simulink model "milestoneone_mdl"  (R2024b)
settings: Solver=FixedStepAuto  StartTime=0.0  StopTime=10  FixedStep=1e-3  RelTol=1e-3  EnableMultiTasking=on
model workspace (MAT data in the model file):
  Var = 0
settings Model: ExtModeTrigDuration=5  Creator=alber  LastModifiedBy=alber
settings OptimizationCC: DefaultParameterBehavior=Inlined  EnhancedBackFolding=on  PassReuseOutputArgsAs=Individual arguments  ZeroExternalMemoryAtStartup=off  ZeroInternalMemoryAtStartup=off  MaxStackSize=64  OptimizeBlockOrder=speed  DifferentSizesBufferReuse=on  OptimizationCustomize=off  EfficientTunableParamExpr=on
settings DebuggingCC: ParameterTunabilityLossMsg=error
settings HardwareCC: ProdBitPerPointer=32  ProdBitPerSizeT=32  ProdBitPerPtrDiffT=32  ProdLargestAtomicInteger=Long  ProdLargestAtomicFloat=Double  ProdWordSize=32  ProdHWDeviceType=ARM Compatible->ARM Cortex
settings SFSimCC: MATLABDynamicMemAlloc=off
settings RTWCC: Description=Embedded Coder  SystemTargetFile=ert.tlc  HardwareBoard=NXP FRDM-K64F  TLCOptions="-aInlineSetEventsForThisBaseRateFcn=TLC_FALSE -aSuppressMultiTaskScheduler=TLC_FALSE  -aRateBasedStepFcn=0"  TemplateMakefile=ert_default_tmf  Toolchain=GNU Tools for ARM Embedded Processors
settings CodeAppCC: ForceParamTrailComments=on  IgnoreCustomStorageClasses=off  OperatorAnnotations=on  SimulinkDataObjDesc=on  SFDataObjDesc=on  InsertBlockDesc=on
settings ERTTargetCC: ExtModeTransport=4  ExtModeMexFile=sendToCommService
settings ConfigComp: CovBoundaryAbsTol=1.0e-5

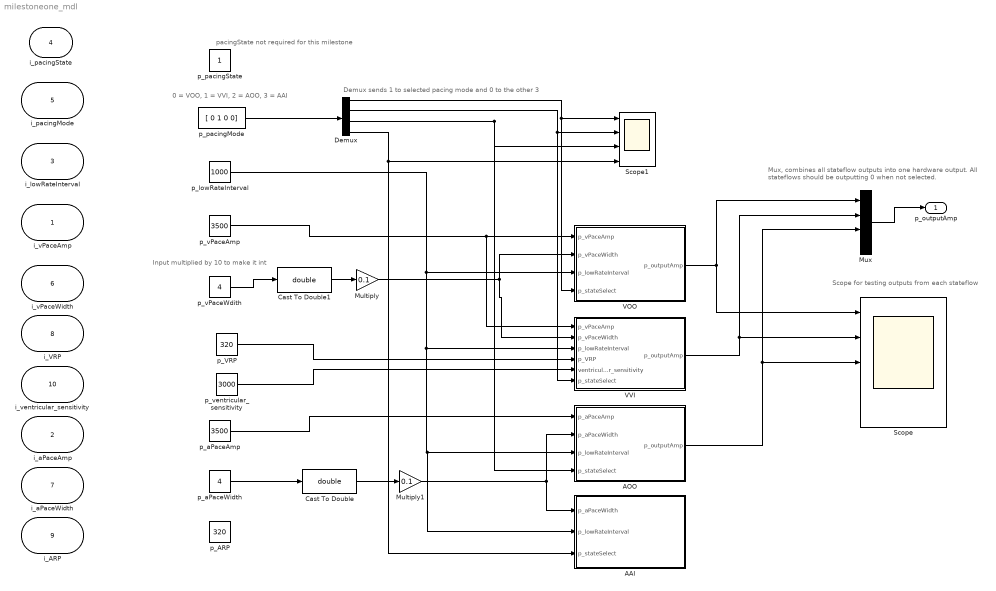
== system milestoneone_mdl ==
  note: pacingState not required for this milestone
  note: Demux sends 1 to selected pacing mode and 0 to the other 3
  note: Input multiplied by 10 to make it int
  note: 0 = VOO, 1 = VVI, 2 = AOO, 3 = AAI
  note: Scope for testing outputs from each stateflow
  note: Mux, combines all stateflow outputs into one hardware output.
      | All stateflows should be outputting 0 when not selected.
  i_vPaceAmp : Inport  OutMin=[500]  OutMax=[7000]  OutDataTypeStr=uint16  Unit=mV  PortDimensions=1
  i_aPaceAmp : Inport  Port=2  OutDataTypeStr=uint16  Unit=mV  PortDimensions=1
  i_lowRateInterval : Inport  Port=3  OutMin=[343]  OutMax=[2000]  OutDataTypeStr=uint16  Unit=Msec  PortDimensions=1
  i_pacingState : Inport  Port=4
  i_pacingMode : Inport  Port=5  OutDataTypeStr=uint8  PortDimensions=1
  i_vPaceWidth : Inport  Port=6  OutMin=1  OutMax=1.9  OutDataTypeStr=uint16  Unit=Msec  PortDimensions=1
  i_aPaceWidth : Inport  Port=7  OutDataTypeStr=uint16  Unit=Msec  PortDimensions=1
  i_VRP : Inport  Port=8  OutMin=[150]  OutMax=[500]  OutDataTypeStr=uint16  Unit=Msec  PortDimensions=1
  i_ARP : Inport  Port=9  OutDataTypeStr=uint16  Unit=mSec  PortDimensions=1
  i_ventricular_sensitivity : Inport  Port=10  OutDataTypeStr=uint16  PortDimensions=1
  AAI : Stateflow chart  TreatAsAtomicUnit=on
  AOO : Stateflow chart  TreatAsAtomicUnit=on
  Cast To Double : DataTypeConversion  OutDataTypeStr=double  SaturateOnIntegerOverflow=off  RndMeth=Floor
  Cast To Double1 : DataTypeConversion  OutDataTypeStr=double  SaturateOnIntegerOverflow=off  RndMeth=Floor
  Demux : Demux
  Multiply : Gain  Gain=0.1
  Multiply1 : Gain  Gain=0.1
  Mux : Mux
  Scope : Scope  NumInputPorts=5
  Scope1 : Scope  NumInputPorts=4
  VOO : Stateflow chart  TreatAsAtomicUnit=on
  VVI : Stateflow chart  TreatAsAtomicUnit=on
  p_ARP : Constant  Value=320  OutDataTypeStr=uint16
  p_VRP : Constant  Value=320  OutMin=[150]  OutMax=[500]  OutDataTypeStr=uint16
  p_aPaceAmp : Constant  Value=3500  OutDataTypeStr=uint16
  p_aPaceWidth : Constant  Value=4  OutDataTypeStr=int16
  p_lowRateInterval : Constant  Value=1000  OutMin=[343]  OutMax=[2000]  OutDataTypeStr=uint16
  p_pacingMode : Constant  Value=[ 0 1 0 0]  OutDataTypeStr=uint8
  p_pacingState : Constant  OutDataTypeStr=uint8
  p_vPaceAmp : Constant  Value=3500  OutMin=[500]  OutMax=[7000]  OutDataTypeStr=uint16
  p_vPaceWdith : Constant  Value=4  OutMin=[1]  OutMax=[19]  OutDataTypeStr=int16
  p_ventricular_sensitivity : Constant  Value=3000  OutDataTypeStr=uint16
  p_outputAmp : Outport
  wires:
  VVI/1(p_outputAmp) -> Mux/2, Scope/2
  AOO/1(p_outputAmp) -> Mux/3, Scope/3
  Mux/1 -> p_outputAmp/1
  Multiply/1 -> VOO/2(p_vPaceWidth), VVI/2(p_vPaceWidth)
  Cast To Double1/1 -> Multiply/1
  Cast To Double/1 -> Multiply1/1
  Multiply1/1 -> AAI/1(p_aPaceWidth), AOO/2(p_aPaceWidth)
  Demux/1 -> Scope1/1, VOO/4(p_stateSelect)
  Demux/2 -> Scope1/2, VVI/6(p_stateSelect)
  Demux/3 -> Scope1/3, AOO/4(p_stateSelect)
  Demux/4 -> AAI/3(p_stateSelect), Scope1/4
  p_pacingMode/1 -> Demux/1
  p_aPaceWidth/1 -> Cast To Double/1
  p_aPaceAmp/1 -> AOO/1(p_aPaceAmp)
  p_lowRateInterval/1 -> AAI/2(p_lowRateInterval), AOO/3(p_lowRateInterval), VVI/3(p_lowRateInterval), VOO/3(p_lowRateInterval)
  p_vPaceAmp/1 -> VVI/1(p_vPaceAmp), VOO/1(p_vPaceAmp)
  p_vPaceWdith/1 -> Cast To Double1/1
  p_VRP/1 -> VVI/4(p_VRP)
  p_ventricular_sensitivity/1 -> VVI/5(ventricular_sensitivity)
  VOO/1(p_outputAmp) -> Scope/1, Mux/1

== stateflow chart milestoneone_mdl/VOO ==
  note: Total cycle time - time already elapsed this cycle
  note: VOO Pacing Mode
  state CHARGE
    entry:
    % Output 0V
    p_outputAmp = 0;
    current_state = "VOO CHARGE"
    % Rest time = total cycle time - pace width
  state PACE
    entry:
    % Output pace at specified amplitude
    p_outputAmp = p_vPaceAmp;
    current_state = "VOO PACE"
    % Wait so that the pace has the specified width
  state INACTIVE
    % Stateflow is inactive when not selected
  CHARGE -> PACE [order 2] : [after(p_lowRateInterval - p_vPaceWidth, msec)]
  (default) -> INACTIVE
  INACTIVE -> CHARGE [order 1] : [p_stateSelect == 1]
  CHARGE -> INACTIVE [order 1] : [p_stateSelect == 0]
  INACTIVE -> INACTIVE [order 2] : [p_stateSelect == 0]
  PACE -> CHARGE : after(p_vPaceWidth, msec)
  data: data local; p_outputAmp output uint16; p_vPaceAmp input uint16 =3500; p_vPaceWidth input double =0.4; p_lowRateInterval input uint16 =6000/low_rate_lim; p_stateSelect input uint8; current_state local string

== stateflow chart milestoneone_mdl/AAI ==
  state PACING
    entry:
    state_out = "AAI PACING"
    AP = true; % deliver pacing pulse
    In_ARP = false;
    timer = 0;
    during:
    timer = timer + 1;
    if (timer >= p_aPaceWidth)
    % Pulse width elapsed -> stop pacing
    AP = false;
    % -> Refractory
    end
  state WAIT
    entry:
    state_out = "AAI WAIT";
    AP = false;
    In_ARP = false;
    timer = 0;
    during:
    if (AS && ~In_ARP)
    % Detected intrinsic atrial beat before timeout
    timer = 0;
    %transition_to(Refractory);
    % ^ Causes an error, add back in later
    elseif (timer >= p_lowRateInterval)
    %Timeout -> no intrinsic beat, deliver pulse
    % ->Pacing
    end
  state INACTIVE
  state Refractory
    entry:
    state_out = "AAI REFRACTORY"
    In_ARP = true;
    AP = false;
    timer = 0;
    during:
    timer = timer + 1;
    % Ignore all AS during ARP
    if (timer >= ARP)
    In_ARP = false;
    timer = 0;
    % -> Waiting
    end
  WAIT -> PACING [order 2] : [timer >= p_lowRateInterval]
  PACING -> Refractory : [after(p_aPaceWidth, msec)]
  (default) -> INACTIVE
  INACTIVE -> WAIT [order 1] : [p_stateSelect == 1]
  WAIT -> INACTIVE [order 1] : [p_stateSelect == 0]
  INACTIVE -> INACTIVE [order 2] : [p_stateSelect == 0]
  WAIT -> Refractory [order 3] : [AS && In_ARP]
  Refractory -> WAIT : [after(ARP, msec)]
  data: data local; data local; p_aPaceWidth input double =0.4; p_lowRateInterval input uint16 =6000/low_rate_lim; AP local boolean =false; In_ARP local boolean =false; ARP local uint16 =0; AS local uint16 =0; timer local uint16 =0; p_stateSelect input; state_out local string

== stateflow chart milestoneone_mdl/VVI ==
  state PACING
    entry:
    current_state = "VVI PACING"
    % Generate pace
    p_outputAmp = p_vPaceAmp;
  note: VVI
  state REFRACTORY
    entry:
    current_state = "VVI REFRACTORY"
    % Stop generating pace
    p_outputAmp = 0;
    % Wait for a refractory period
  note: Stateflow cycles in INACTIVE when not selected
  state SENSING
    entry:
    current_state = "VVI SENSING"
    % If the input signal is higher than the
    % sensitivity threshold, wait for another
    % refractory period
    % If the low rate interval passes and no
    % signals higher than the threshold are
    % detected, send another pace
  state INACTIVE
    % When stateflow isn't selected
  PACING -> REFRACTORY : [after(p_vPaceWidth, msec)]
  (default) -> INACTIVE
  SENSING -> REFRACTORY [order 3] : [p_vPaceAmp >= ventricular_sensitivity]
  SENSING -> PACING [order 2] : [after(p_lowRateInterval, msec)]
  REFRACTORY -> SENSING : [after(p_VRP, msec)]
  INACTIVE -> SENSING [order 1] : [p_stateSelect == 1]
  SENSING -> INACTIVE [order 1] : [p_stateSelect == 0]
  INACTIVE -> INACTIVE [order 2] : [p_stateSelect == 0]
  data: p_vPaceAmp input uint16 =3500; p_vPaceWidth input double =0.4; p_lowRateInterval input uint16 =6000/low_rate_lim; output_pulse_flag local double; pacing_done_flag local double; p_VRP input uint16; ventricular_sensitivity input uint16; p_outputAmp output uint16; p_stateSelect input uint8; current_state local string

== stateflow chart milestoneone_mdl/AOO ==
  note: Max total cycle time - time already elapsed this cycle
  note: AOO Pacing Mode
  note: Cycle through this state when AoO isn't selected
  state PACE
    entry:
    %Send out pace signal
    p_outputAmp = p_aPaceAmp;
    current_state = "AOO PACE"
    % Wait for the width of a pace
  state CHARGE
    entry:
    % Stop pacing, wait rest of cycle time
    p_outputAmp = 0;
    current_state = "AOO CHARGE"
  state INACTIVE
    % When state is not selected by input
  CHARGE -> PACE [order 2] : [after(p_lowRateInterval - p_aPaceWidth, msec)]
  (default) -> INACTIVE
  INACTIVE -> CHARGE [order 1] : [p_stateSelect == 1]
  CHARGE -> INACTIVE [order 1] : [p_stateSelect == 0]
  INACTIVE -> INACTIVE [order 2] : [p_stateSelect == 0]
  PACE -> CHARGE : after(p_aPaceWidth, msec)
  data: data local; p_outputAmp output uint16; p_aPaceAmp input uint16 =3500; p_aPaceWidth input double =0.4; p_lowRateInterval input uint16 =6000/low_rate_lim; output_pace_flag local boolean; p_stateSelect input uint8; current_state local string
